simulink model "HbridgeInverter"  (R2023b)
settings: Solver=VariableStepAuto  StartTime=0.0  StopTime=0.1  RelTol=1e-3
libraries: spsMosfetLib x4, spsSeriesRLCBranchLib x3, spsCurrentMeasurementLib x2, spsVoltageMeasurementLib x2, spsDCVoltageSourceLib x1, spsPWMGeneratorDCDCLib x1, eePowerMeasurement x1, sps_lib x1
settings Model: Creator=mukoo  LastModifiedBy=mukoo
settings DataIOCC: ReturnWorkspaceOutputs=off

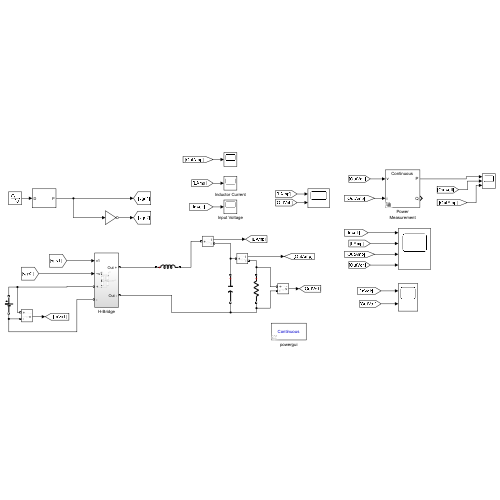
[thumbnail: Simulink's stored preview of the top-level diagram]
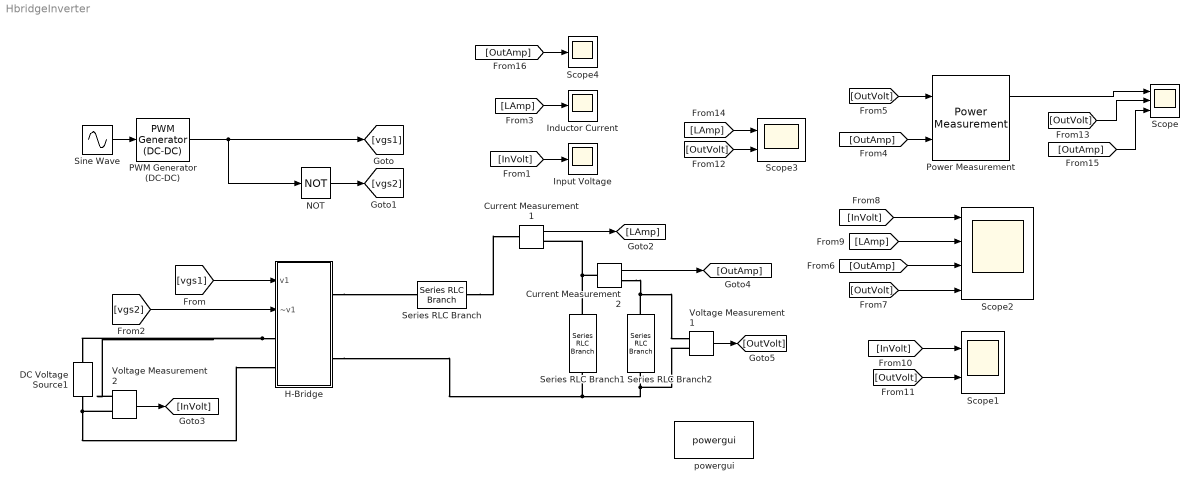
== system HbridgeInverter ==
  Current Measurement1 : spsCurrentMeasurementLib/Current Measurement  PhasorSimulation=off  OutputType=Complex  PSBequivalent=0
  Current Measurement2 : spsCurrentMeasurementLib/Current Measurement  PhasorSimulation=off  OutputType=Complex  PSBequivalent=0
  DC Voltage Source1 : spsDCVoltageSourceLib/DC Voltage Source  Amplitude=35  Measurements=None
  H-Bridge : Subsystem
  Inductor Current : Scope
  Input Voltage : Scope
  NOT : Logic  Operator=NOT  IconShape=distinctive  AllPortsSameDT=off  OutDataTypeStr=boolean
  PWM Generator (DC-DC) : spsPWMGeneratorDCDCLib/PWM Generator (DC-DC)  Fsw=25000  Ts=0
  Power Measurement : eePowerMeasurement/Power Measurement  LabelModeActiveChoice=Continuous  F=2*pi*60  K=0  Ts=0
  Scope : Scope  NumInputPorts=3
  Scope1 : Scope  NumInputPorts=2
  Scope2 : Scope  NumInputPorts=4
  Scope3 : Scope  NumInputPorts=2
  Scope4 : Scope
  Series RLC Branch : spsSeriesRLCBranchLib/Series RLC Branch  LConnTagsString=__new0  RConnTagsString=__new0  BranchType=L  Resistance=1  Inductance=1e-3  SetiL0=off  InitialCurrent=0  Capacitance=1e-6  Setx0=off  InitialVoltage=0  Measurements=None
  Series RLC Branch1 : spsSeriesRLCBranchLib/Series RLC Branch  LConnTagsString=__new0  RConnTagsString=__new0  BranchType=C  Resistance=1  Inductance=1e-3  SetiL0=off  InitialCurrent=0  Capacitance=20e-6  Setx0=off  InitialVoltage=0  Measurements=None
  Series RLC Branch2 : spsSeriesRLCBranchLib/Series RLC Branch  LConnTagsString=__new0  RConnTagsString=__new0  BranchType=R  Resistance=3  Inductance=1e-3  SetiL0=off  InitialCurrent=0  Capacitance=1e-6  Setx0=off  InitialVoltage=0  Measurements=None
  Sine Wave : Sin  Amplitude=0.5  Bias=0.5  Frequency=2*pi*60  SampleTime=0
  Voltage Measurement1 : spsVoltageMeasurementLib/Voltage Measurement  PhasorSimulation=off  OutputType=Complex  PSBequivalent=0
  Voltage Measurement2 : spsVoltageMeasurementLib/Voltage Measurement  PhasorSimulation=off  OutputType=Complex  PSBequivalent=0
  powergui : sps_lib/powergui  Priority=1  SimulationMode=Continuous  SampleTime=50e-6  frequency=60  Iterations=50  frequencyindice=0  Pbase=100e6  ErrMax=1e-4  UnitsV=kV  UnitsW=MW  buscounter=0  FunctionMessages=off  echomessages=off  EnableUseOfTLC=off  CurrentSourceSwitches=off  DisableSnubberDevices=off  DisableRonSwitches=off  DisableVfSwitches=off  DisplayEquations=off  AutomaticDiscreteSolvers=off  SolverType=Tustin/Backward Euler (TBE)  Interpol=off  ExternalGateDelay=off  methode=off  Ts=100  x0status=blocks  SPID=on  SwTol=0  HookPort=off  NonlinearTolerance=1e-4  nMaxIteration=100  ContinueOnMaxIteration=off  RestoreLinks=warning  ResistiveCurrentMeasurement=off  Frange=[0:2:500]  Ylog=off  Xlog=on  ShowGrid=off  save=off  variable=ZData  structure=0  ZoomFFT=off  StartTime=0.0  cycles=1  DisplayStyle=1  fundamental=60  FreqAxis=off  MaxFrequency=1000  frequencyindicesteady=1  RmsSteady=1  display=off
  wires:
  PWM Generator (DC-DC)/1 -> [vgs1], NOT/1
  Sine Wave/1 -> PWM Generator (DC-DC)/1
  Current Measurement1/1 -> [LAmp]
  Voltage Measurement1/1 -> [OutVolt]
  NOT/1 -> [vgs2]
  [vgs1] -> H-Bridge/1(v1)
  [vgs2] -> H-Bridge/2(~v1)
  Voltage Measurement2/1 -> [InVolt]
  Current Measurement2/1 -> [OutAmp]
  [InVolt] -> Input Voltage/1
  [LAmp] -> Inductor Current/1
  [OutAmp] -> Power Measurement/2
  [OutVolt] -> Power Measurement/1
  [OutAmp] -> Scope2/3
  [OutVolt] -> Scope2/4
  [InVolt] -> Scope2/1
  [LAmp] -> Scope2/2
  [InVolt] -> Scope1/1
  [OutVolt] -> Scope1/2
  Power Measurement/1 -> Scope/1
  [LAmp] -> Scope3/1
  [OutVolt] -> Scope3/2
  [OutVolt] -> Scope/2
  [OutAmp] -> Scope/3
  [OutAmp] -> Scope4/1
  connections:
  DC Voltage Source1/LConn1 -- H-Bridge/LConn2 -- Voltage Measurement2/LConn2
  Series RLC Branch1/LConn1 -- Current Measurement2/LConn1 -- Current Measurement1/RConn1
  Series RLC Branch/RConn1 -- Current Measurement1/LConn1
  Series RLC Branch2/LConn1 -- Current Measurement2/RConn1 -- Voltage Measurement1/LConn1
  H-Bridge/RConn2 -- Series RLC Branch1/RConn1 -- Voltage Measurement1/LConn2 -- Series RLC Branch2/RConn1
  H-Bridge/RConn1 -- Series RLC Branch/LConn1
  H-Bridge/LConn1 -- DC Voltage Source1/RConn1 -- Voltage Measurement2/LConn1

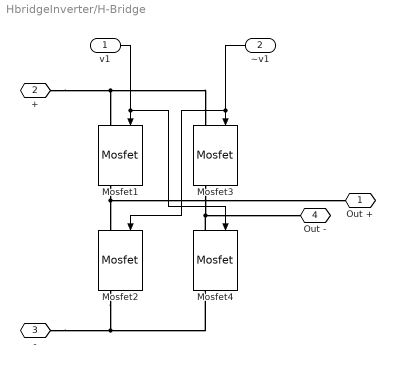
== system HbridgeInverter/H-Bridge ==
  v1 : Inport
  ~v1 : Inport  Port=2
  Mosfet{1..4} (4 alike) : spsMosfetLib/Mosfet  Ron=0.1  Lon=0  Rd=0.01  Vfd=0  IC=0  Rs=1e5  Cs=inf  Measurements=on
  Out + : PMIOPort  Side=Right
  + : PMIOPort  Port=2  Side=Left
  - : PMIOPort  Port=3  Side=Left
  Out - : PMIOPort  Port=4  Side=Right
  wires:
  ~v1/1 -> Mosfet2/1, Mosfet3/1
  v1/1 -> Mosfet4/1, Mosfet1/1
  connections:
  Mosfet1/RConn1 -- Out +/RConn1 -- Mosfet2/LConn1
  Mosfet2/RConn1 -- -/RConn1 -- Mosfet4/RConn1
  Mosfet4/LConn1 -- Out -/RConn1 -- Mosfet3/RConn1
  Mosfet3/LConn1 -- Mosfet1/LConn1 -- +/RConn1
